simulink model "SOFC_smlkCH4"  (R2015b)
settings: Solver=ode113  SolverMode=SingleTasking  StartTime=0.0  StopTime=1000  MaxStep=1  MinStep=0.00001  RelTol=1e-3
values from neighbouring files (symbols this model uses):
  A_an = 1.05e-05    [SOFC_CH4data.m]    (also in SOFC_H2data.m)
  A_cat = 2.38e-05    [SOFC_CH4data.m]    (also in SOFC_H2data.m)
  A_cell = 180    [SOFC_begin.m]
  A_el = 0.03 / T    [SOFC_CH4data.m]    (also in SOFC_H2data.m)
  B_an = -1150    [SOFC_CH4data.m]    (also in SOFC_H2data.m)
  B_cat = 1200    [SOFC_CH4data.m]    (also in SOFC_H2data.m)
  B_el = 10300    [SOFC_CH4data.m]    (also in SOFC_H2data.m)
  c_cw = 4.18e03    (= 4180)    [SOFC_CH4data.m]    (also in SOFC_H2data.m)
  C_th = 500e03    (= 500000)    [SOFC_CH4data.m]    (also in SOFC_H2data.m)
  CV = nH2_FCin_ / n_fuel    [SOFC_CH4data.m]
  CV_H2O = nH2O_FCin_ / n_fuel    [SOFC_CH4data.m]
  E_act_an = 75e03    (= 75000)    [SOFC_CH4data.m]    (also in SOFC_H2data.m)
  E_act_cat = 96e03    (= 96000)    [SOFC_CH4data.m]    (also in SOFC_H2data.m)
  eta_ACDC = 0.90    (= 0.9)    [SOFC_CH4data.m]    (also in SOFC_H2data.m = 0.95)
  eta_comb = 0.95    [SOFC_CH4data.m]    (also in SOFC_H2data.m = 1)
  eta_hx = 0.90    (= 0.9)    [SOFC_CH4data.m]    (also in SOFC_H2data.m = 0.92)
  F = 96485    [SOFC_begin.m]
  F_airsplit = 2.0    (= 2)    [SOFC_CH4data.m]    (also in SOFC_H2data.m = 1.1)
  F_pr = 3.0711    [SOFC_CH4data.m]
  gamma_an = 5.5e4    (= 55000)    [SOFC_CH4data.m]    (also in SOFC_H2data.m)
  gamma_cat = 7.0e4    (= 70000)    [SOFC_CH4data.m]    (also in SOFC_H2data.m)
  h_airc = gamma_air * R * T / (gamma_air - 1) * ((1 / beta_c)^     ((gamma_air - 1) / gamma_air) - 1) / eta_c    [SOFC_CH4data.m]    (also in SOFC_H2data.m)
  h_airpc = (h_aircomb - h_airexh) / 1000 * M_air    [SOFC_CH4data.m]    (also in SOFC_H2data.m)
  h_airpr = (hairpr_out - hairpr_in) * M_air / eta_ph    [SOFC_CH4data.m]
  h_Arpc = (h_Arcomb - h_Arexh) / 1000 * M_Ar    [SOFC_CH4data.m]    (also in SOFC_H2data.m)
  h_CH4c = gamma_CH4 * R * T / (gamma_CH4 - 1) * ((1 / beta_c)^     ((gamma_CH4 - 1) / gamma_CH4) - 1) / eta_c    [SOFC_CH4data.m]
  h_CH4ref = -206000    [SOFC_CH4data.m]
  h_CO2pc = (h_CO2comb - h_CO2exh) / 1000 * M_CO2    [SOFC_CH4data.m]    (also in SOFC_H2data.m)
  h_cond = 500    [SOFC_CH4data.m]    (also in SOFC_H2data.m)
  h_conv = 0.1    [SOFC_CH4data.m]    (also in SOFC_H2data.m)
  h_COpc = C_COcomb * (Tcomb - Texh) * M_CO    (= 23740.08)    [SOFC_CH4data.m]
  h_fpr = (hfpr_out - hfpr_in) / eta_ph    [SOFC_CH4data.m]
  h_H2Opc = C_H2Ocomb * (Tcomb - Texh) / 1000 * M_H2O    [SOFC_CH4data.m]    (also in SOFC_H2data.m)
  h_H2Opcvap = WaterEnthalpyVaporization (pcomb/101325, Texh)    [SOFC_CH4data.m]    (also in SOFC_H2data.m)
  h_H2Opr = ((hH2Opr_out - hH2Opr_in) * M_H2O + h_H2Oprv) / eta_ph    [SOFC_CH4data.m]
  h_H2pc = C_H2comb * (Tcomb - Texh) / 1000 * M_H2    [SOFC_CH4data.m]    (also in SOFC_H2data.m)
  h_N2pc = (h_N2comb - h_N2exh) / 1000 * M_N2    [SOFC_CH4data.m]    (also in SOFC_H2data.m)
  h_O2pc = (h_O2comb - h_O2exh) / 1000 * M_O2    [SOFC_CH4data.m]    (also in SOFC_H2data.m)
  i_max = 0.88    [SOFC_CH4data.m]    (also in SOFC_H2data.m)
  K_H2 = 8.34e-01    (= 0.834)    [SOFC_CH4data.m]    (also in SOFC_H2data.m)
  K_H2O = 2.81e-01    (= 0.281)    [SOFC_CH4data.m]    (also in SOFC_H2data.m)
  K_O2 = 2.52e-00    (= 2.52)    [SOFC_CH4data.m]    (also in SOFC_H2data.m)
  K_r = N_cell / (4 * F)    [SOFC_CH4data.m]    (also in SOFC_H2data.m)
  lambda = 9.15    [SOFC_begin.m]
  m_cw = 0.25000    (= 0.25)    [SOFC_CH4data.m]    (also in SOFC_H2data.m)
  N_cell = 38    [SOFC_begin.m]
  p_atm = 1.01325e05    (= 101325)    [SOFC_begin.m]
  P_gamma = 190.0    (= 190)    [SOFC_CH4data.m]    (also in SOFC_H2data.m = 100)
  p_H20 = pp_fin(6) / 101325    [SOFC_CH4data.m]    (also in SOFC_H2data.m = y_H2in * p_an / 101325)
  p_H2O0 = pp_fin(7) / 101325    [SOFC_CH4data.m]    (also in SOFC_H2data.m = y_H2Oin * p_an / 101325)
  p_O20 = pp_ain(5) / 101325    [SOFC_CH4data.m]    (also in SOFC_H2data.m = x_O2in * p_cat / 101325)
  Q_COref = n_COref * h_COref    [SOFC_CH4data.m]
  Q_gamma = 0.0    (= 0)    [SOFC_CH4data.m]    (also in SOFC_H2data.m = 30)
  R = P_SOFC ./ (P_SOFC ./ etae_aux .* etat)    [SOFC_begin.m]
  R_th = 0.0817    [SOFC_CH4data.m]    (also in SOFC_H2data.m)
  SC = 2.16    [SOFC_CH4data.m]
  T = 750 + 273.15    (= 1023.15)    [SOFC_begin.m]
  T0 = T_a    [SOFC_CH4data.m]    (also in SOFC_H2data.m)
  T_a = 25    [SOFC_begin.m]
  t_an = 0.0545    [SOFC_CH4data.m]    (also in SOFC_H2data.m)
  t_cat = 0.004    [SOFC_CH4data.m]    (also in SOFC_H2data.m)
  T_cwin = 20 + 0    (= 20)    [SOFC_CH4data.m]    (also in SOFC_H2data.m)
  T_des = T - 273.15    [SOFC_CH4data.m]    (also in SOFC_H2data.m)
  t_el = 0.0005    [SOFC_CH4data.m]    (also in SOFC_H2data.m)
  tau1_ref = 2    [SOFC_CH4data.m]
  tau2_ref = 2    [SOFC_CH4data.m]
  tau_H2 = 26.1    [SOFC_CH4data.m]    (also in SOFC_H2data.m)
  tau_H2O = 78.30    (= 78.3)    [SOFC_CH4data.m]    (also in SOFC_H2data.m)
  tau_hx = 15.0    (= 15)    [SOFC_CH4data.m]    (also in SOFC_H2data.m)
  tau_O2 = 2.91    [SOFC_CH4data.m]    (also in SOFC_H2data.m)
  tau_ph = 5.00    (= 5)    [SOFC_CH4data.m]    (also in SOFC_H2data.m)
  tau_th = C_th * R_th    (= 40850)    [SOFC_CH4data.m]    (also in SOFC_H2data.m)
  theta = 0.910    (= 0.91)    [SOFC_CH4data.m]    (also in SOFC_H2data.m)
  U = polyval(polU, n_CH4in(1))    [SOFC_CH4data.m]    (also in SOFC_H2data.m = polyval(polU, n_H2in(1)))
  V_tn = 1.48    [SOFC_CH4data.m]    (also in SOFC_H2data.m)
  x_Ar = 0.0092    [SOFC_begin.m]
  x_CO2 = 0.0004    [SOFC_begin.m]
  x_H2O = 0.0103    [SOFC_begin.m]
  x_H2Ovap = WaterSaturationPressure (Texh) / (pcomb/101325)    [SOFC_CH4data.m]    (also in SOFC_H2data.m)
  x_N2 = 0.7728    [SOFC_begin.m]
  x_O2 = 0.2073    [SOFC_begin.m]
  xi1 = n_fuel * yy_in(1)    [SOFC_CH4data.m]    (also in SOFC_cellstack.m = n_a * yy(1))
  xi2 = n_fuel * (yy_in(1) + yy_in(2)) * 0.92    [SOFC_CH4data.m]    (also in SOFC_cellstack.m = xi)
  xi3 = U * n_fuel * (4 * yy_in(1) + yy_in(2) + yy_in(6))    [SOFC_CH4data.m]    (also in SOFC_cellstack.m = U * n_a * (4 * yy(1) + yy(2) + yy(6)))
  xi4 = nn_fout(6) * eta_comb    [SOFC_CH4data.m]    (also in SOFC_H2data.m = n_H2out * eta_comb)
  xi5 = nn_fout(2) * eta_comb    [SOFC_CH4data.m]
  y_CH4 = 0.2832    [SOFC_begin.m]
  y_CO = 0.0207    [SOFC_begin.m]
  y_CO2 = 0    [SOFC_begin.m]
  y_H2 = 0.0482    [SOFC_begin.m]
  y_H2O = 0.6348    [SOFC_begin.m]
  y_N2 = 0.0131    [SOFC_begin.m]
undefined symbols (not defined in the file or in its folder): magnitude
settings Model: Creator=gapaolo  LastModifiedBy=gapaolo
settings DataIOCC: SaveFormat=Array
settings OptimizationCC: BlockReduction=off  BooleanDataType=off
settings DebuggingCC: AlgebraicLoopMsg=none  SaveWithParameterizedLinksMsg=none  UnderspecifiedInitializationDetection=Classic  MergeDetectMultiDrivingBlocksExec=none  SignalResolutionControl=TryResolveAllWithWarning
settings HardwareCC: ProdBitPerPointer=32  ProdLargestAtomicFloat=None  ProdIntDivRoundTo=Undefined  ProdEndianess=Unspecified  ProdWordSize=32  ProdHWDeviceType=32-bit Generic  TargetUnknown=on
settings GRTTargetCC: GeneratePreprocessorConditionals=Disable all
settings ConfigComp: CovModelRefEnable=Off  CovSFcnEnable=off

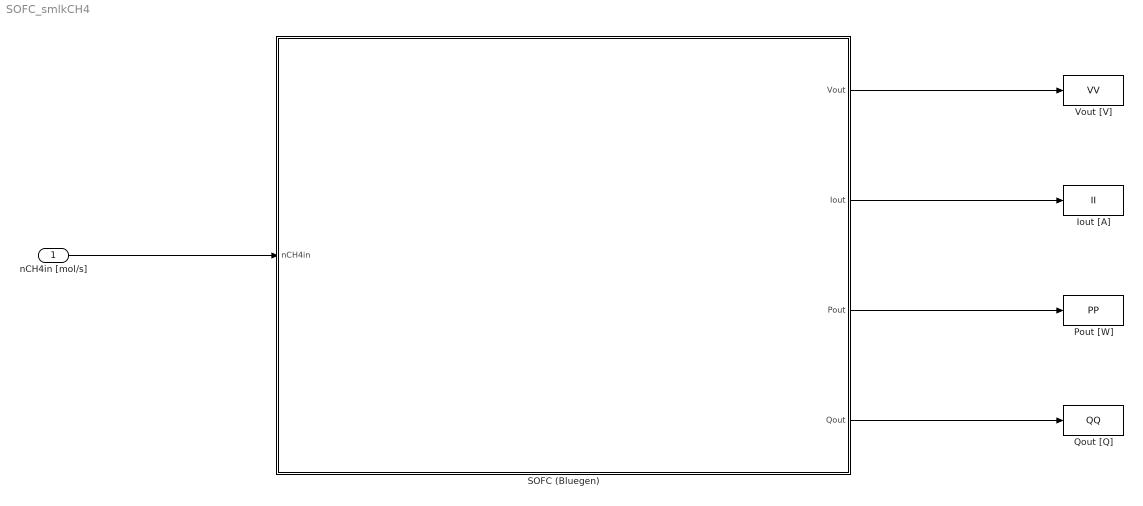
== system SOFC_smlkCH4 ==
  nCH4in [mol/s] : Inport
  Iout [A] : ToWorkspace  VariableName=II  SaveFormat=Timeseries  SampleTime=-1
  Pout [W] : ToWorkspace  VariableName=PP  SaveFormat=Timeseries  SampleTime=-1
  Qout [Q] : ToWorkspace  VariableName=QQ  SaveFormat=Timeseries  SampleTime=-1
  SOFC (Bluegen) : Subsystem
  Vout [V] : ToWorkspace  VariableName=VV  SaveFormat=Timeseries  SampleTime=-1
  wires:
  nCH4in [mol/s]/1 -> SOFC (Bluegen)/1(nCH4in)
  SOFC (Bluegen)/1(Vout) -> Vout [V]/1
  SOFC (Bluegen)/2(Iout) -> Iout [A]/1
  SOFC (Bluegen)/3(Pout) -> Pout [W]/1
  SOFC (Bluegen)/4(Qout) -> Qout [Q]/1

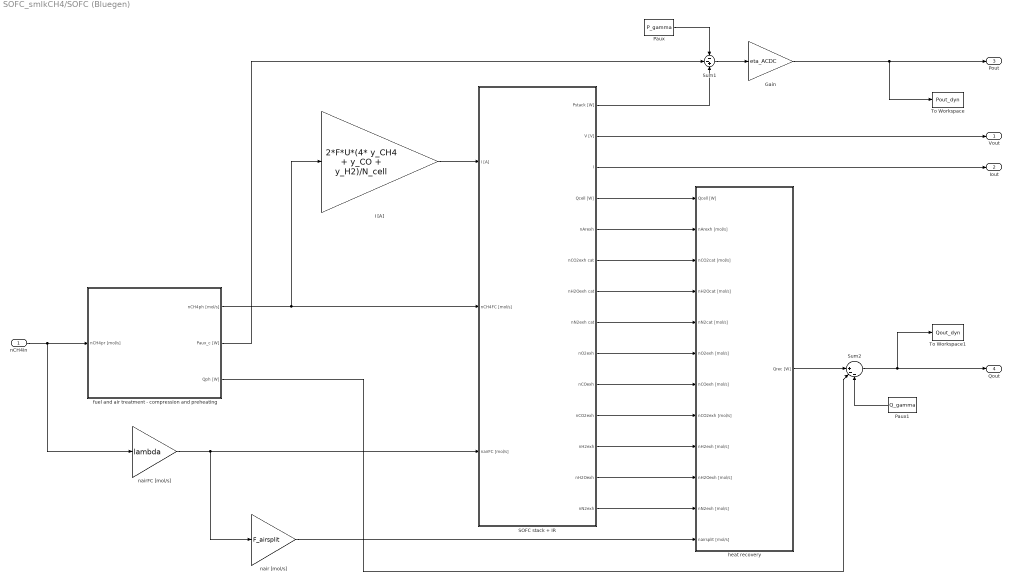
== system SOFC_smlkCH4/SOFC (Bluegen) ==
  nCH4in : Inport
  Gain : Gain  Gain=eta_ACDC
  I [A] : Gain  Gain=2*F*U*(4* y_CH4 + y_CO + y_H2)/N_cell
  Paux : Constant  Value=P_gamma
  Paux1 : Constant  Value=Q_gamma
  SOFC stack + IR : Subsystem
  Sum1 : Sum  Inputs=--+
  Sum2 : Sum  Inputs=||+--
  To Workspace : ToWorkspace  VariableName=Pout_dyn  SaveFormat=Timeseries  SampleTime=-1
  To Workspace1 : ToWorkspace  VariableName=Qout_dyn  SaveFormat=Timeseries  SampleTime=-1
  fuel and air treatment - compression and preheating : Subsystem
  heat recovery : Subsystem
  nair [mol/s] : Gain  Gain=F_airsplit
  nairFC [mol/s] : Gain  Gain=lambda
  Vout : Outport
  Iout : Outport  Port=2
  Pout : Outport  Port=3
  Qout : Outport  Port=4
  wires:
  nCH4in/1 -> fuel and air treatment - compression and preheating/1(nCH4pr [mol/s]), nairFC [mol/s]/1
  fuel and air treatment - compression and preheating/1(nCH4ph [mol/s]) -> I [A]/1, SOFC stack + IR/2(nCH4FC [mol/s])
  I [A]/1 -> SOFC stack + IR/1(I [A])
  nairFC [mol/s]/1 -> nair [mol/s]/1, SOFC stack + IR/3(nairFC [mol/s])
  SOFC stack + IR/4(Qcell [W]) -> heat recovery/1(Qcell [W])
  SOFC stack + IR/5(nArexh) -> heat recovery/2(nArexh [mol/s])
  SOFC stack + IR/6(nCO2exh cat) -> heat recovery/3(nCO2cat [mol/s])
  SOFC stack + IR/7(nH2Oexh cat) -> heat recovery/4(nH2Ocat [mol/s])
  SOFC stack + IR/8(nN2exh cat) -> heat recovery/5(nN2cat [mol/s])
  SOFC stack + IR/9(nO2exh) -> heat recovery/6(nO2exh [mol/s])
  SOFC stack + IR/11(nCO2exh) -> heat recovery/8(nCO2exh [mol/s])
  SOFC stack + IR/12(nH2exh) -> heat recovery/9(nH2exh [mol/s])
  SOFC stack + IR/13(nH2Oexh) -> heat recovery/10(nH2Oexh [mol/s])
  nair [mol/s]/1 -> heat recovery/12(nairsplit [mol/s])
  SOFC stack + IR/10(nCOexh) -> heat recovery/7(nCOexh [mol/s])
  SOFC stack + IR/14(nN2exh) -> heat recovery/11(nN2exh [mol/s])
  SOFC stack + IR/2(V [V]) -> Vout/1
  SOFC stack + IR/3("I ") -> Iout/1
  Sum1/1 -> Gain/1
  SOFC stack + IR/1(Pstack [W]) -> Sum1/3
  fuel and air treatment - compression and preheating/2(Paux_c [W]) -> Sum1/2
  Paux/1 -> Sum1/1
  heat recovery/1(Qrec [W]) -> Sum2/1
  Sum2/1 -> Qout/1, To Workspace1/1
  Gain/1 -> To Workspace/1, Pout/1
  fuel and air treatment - compression and preheating/3(Qph [W]) -> Sum2/2
  Paux1/1 -> Sum2/3

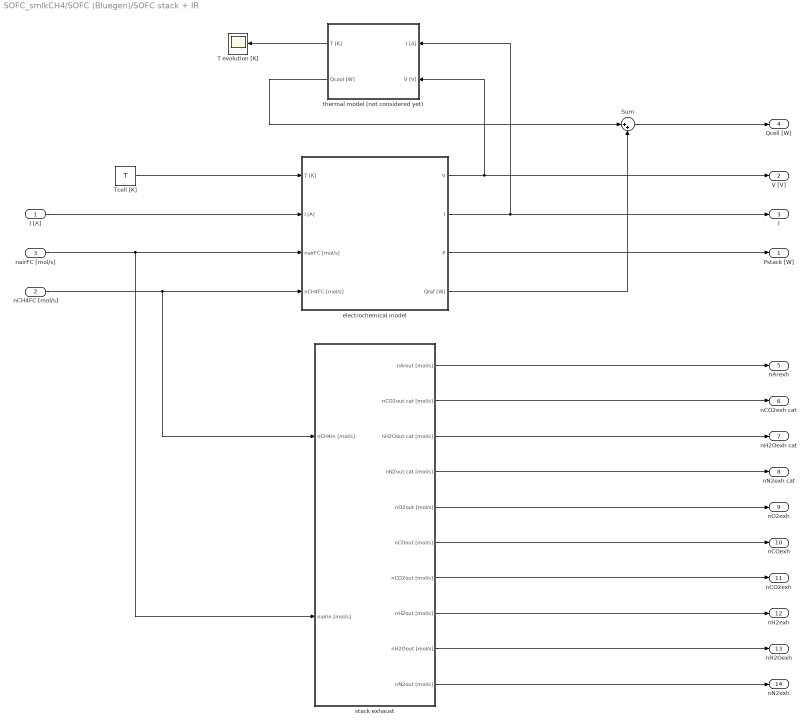
== system SOFC_smlkCH4/SOFC (Bluegen)/SOFC stack + IR ==
  I [A] : Inport
  nCH4FC [mol/s] : Inport  Port=2
  nairFC [mol/s] : Inport  Port=3
  Sum : Sum  Inputs=|++
  T evolution [K] : Scope
  Tcell [K] : Constant  Value=T
  electrochemical model : Subsystem
  stack exhaust : Subsystem
  thermal model (not considered yet) : Subsystem
  Pstack [W] : Outport
  V [V] : Outport  Port=2
  "I " : Outport  Port=3
  Qcell [W] : Outport  Port=4
  nArexh : Outport  Port=5
  nCO2exh cat : Outport  Port=6
  nH2Oexh cat : Outport  Port=7
  nN2exh cat : Outport  Port=8
  nO2exh : Outport  Port=9
  nCOexh : Outport  Port=10
  nCO2exh : Outport  Port=11
  nH2exh : Outport  Port=12
  nH2Oexh : Outport  Port=13
  nN2exh : Outport  Port=14
  wires:
  I [A]/1 -> electrochemical model/2(I [A])
  nairFC [mol/s]/1 -> stack exhaust/2(nairin [mol/s]), electrochemical model/3(nairFC [mol/s])
  nCH4FC [mol/s]/1 -> stack exhaust/1(nCH4in [mol/s]), electrochemical model/4(nCH4FC [mol/s])
  electrochemical model/1(V) -> thermal model (not considered yet)/2(V [V]), V [V]/1
  electrochemical model/2(I) -> "I "/1, thermal model (not considered yet)/1(I [A])
  thermal model (not considered yet)/1(T [K]) -> T evolution [K]/1
  thermal model (not considered yet)/2(Qcool [W]) -> Sum/1
  electrochemical model/3(P) -> Pstack [W]/1
  Tcell [K]/1 -> electrochemical model/1(T [K])
  electrochemical model/4(Qref [W]) -> Sum/2
  Sum/1 -> Qcell [W]/1
  stack exhaust/10(nN2out [mol/s]) -> nN2exh/1
  stack exhaust/9(nH2Oout [mol/s]) -> nH2Oexh/1
  stack exhaust/8(nH2out [mol/s]) -> nH2exh/1
  stack exhaust/7(nCO2out [mol/s]) -> nCO2exh/1
  stack exhaust/6(nCOout [mol/s]) -> nCOexh/1
  stack exhaust/5(nO2out [mol/s]) -> nO2exh/1
  stack exhaust/4(nN2out cat [mol/s]) -> nN2exh cat/1
  stack exhaust/3(nH2Oout cat [mol/s]) -> nH2Oexh cat/1
  stack exhaust/2(nCO2out cat [mol/s]) -> nCO2exh cat/1
  stack exhaust/1(nArout [mol/s]) -> nArexh/1

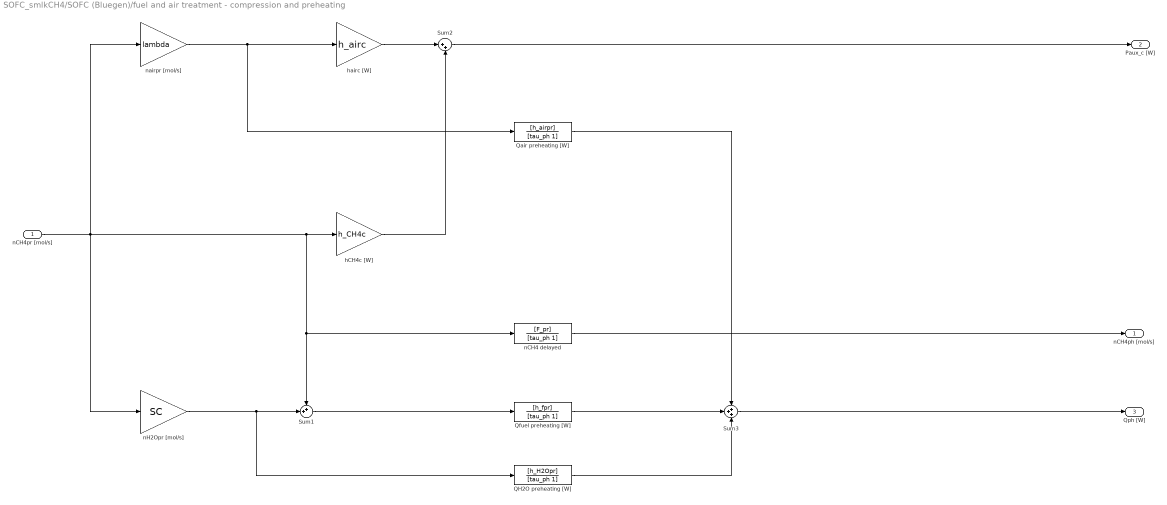
== system SOFC_smlkCH4/SOFC (Bluegen)/fuel and air treatment - compression and preheating ==
  nCH4pr [mol/s] : Inport
  QH2O preheating [W] : TransferFcn  Numerator=[h_H2Opr]  Denominator=[tau_ph 1]
  Qair preheating [W] : TransferFcn  Numerator=[h_airpr]  Denominator=[tau_ph 1]
  Qfuel preheating [W] : TransferFcn  Numerator=[h_fpr]  Denominator=[tau_ph 1]
  Sum1 : Sum  Inputs=++|
  Sum2 : Sum  Inputs=|++
  Sum3 : Sum  Inputs=+++
  hCH4c [W] : Gain  Gain=h_CH4c
  hairc [W] : Gain  Gain=h_airc
  nCH4 delayed : TransferFcn  Numerator=[F_pr]  Denominator=[tau_ph 1]
  nH2Opr [mol/s] : Gain  Gain=SC
  nairpr [mol/s] : Gain  Gain=lambda
  nCH4ph [mol/s] : Outport
  Paux_c [W] : Outport  Port=2
  Qph [W] : Outport  Port=3
  wires:
  nCH4pr [mol/s]/1 -> hCH4c [W]/1, nCH4 delayed/1, Sum1/1, nairpr [mol/s]/1, nH2Opr [mol/s]/1
  nH2Opr [mol/s]/1 -> QH2O preheating [W]/1, Sum1/2
  nairpr [mol/s]/1 -> Qair preheating [W]/1, hairc [W]/1
  hairc [W]/1 -> Sum2/1
  hCH4c [W]/1 -> Sum2/2
  Sum2/1 -> Paux_c [W]/1
  Sum1/1 -> Qfuel preheating [W]/1
  Qfuel preheating [W]/1 -> Sum3/2
  QH2O preheating [W]/1 -> Sum3/3
  Sum3/1 -> Qph [W]/1
  nCH4 delayed/1 -> nCH4ph [mol/s]/1
  Qair preheating [W]/1 -> Sum3/1

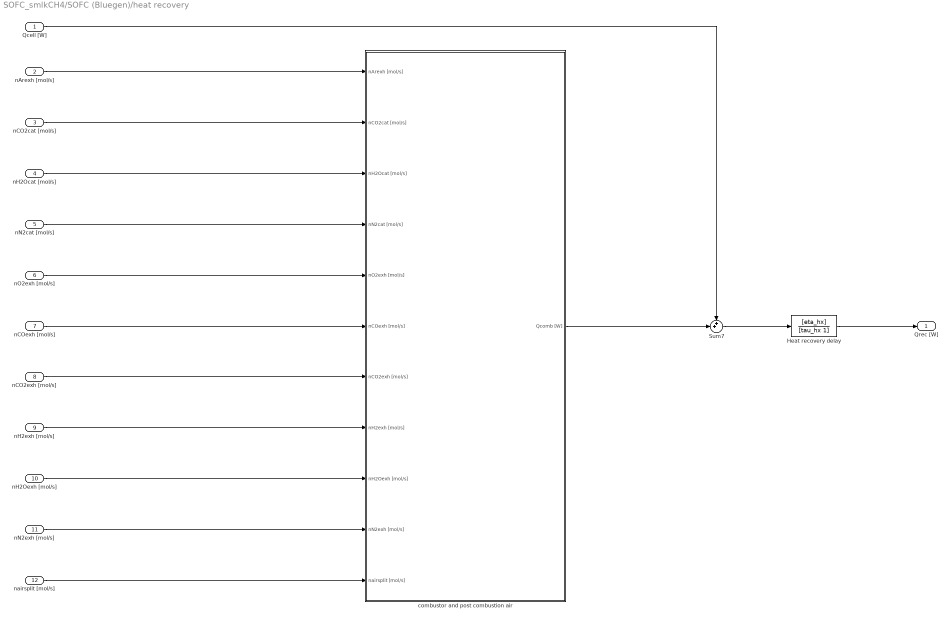
== system SOFC_smlkCH4/SOFC (Bluegen)/heat recovery ==
  Qcell [W] : Inport
  nArexh [mol/s] : Inport  Port=2
  nCO2cat [mol/s] : Inport  Port=3
  nH2Ocat [mol/s] : Inport  Port=4
  nN2cat [mol/s] : Inport  Port=5
  nO2exh [mol/s] : Inport  Port=6
  nCOexh [mol/s] : Inport  Port=7
  nCO2exh [mol/s] : Inport  Port=8
  nH2exh [mol/s] : Inport  Port=9
  nH2Oexh [mol/s] : Inport  Port=10
  nN2exh [mol/s] : Inport  Port=11
  nairsplit [mol/s] : Inport  Port=12
  Heat recovery delay : TransferFcn  Numerator=[eta_hx]  Denominator=[tau_hx 1]
  Sum7 : Sum  Inputs=++|
  combustor and post combustion air : Subsystem
  Qrec [W] : Outport
  wires:
  Heat recovery delay/1 -> Qrec [W]/1
  nArexh [mol/s]/1 -> combustor and post combustion air/1(nArexh [mol/s])
  nCO2cat [mol/s]/1 -> combustor and post combustion air/2(nCO2cat [mol/s])
  nH2Ocat [mol/s]/1 -> combustor and post combustion air/3(nH2Ocat [mol/s])
  nN2cat [mol/s]/1 -> combustor and post combustion air/4(nN2cat [mol/s])
  nO2exh [mol/s]/1 -> combustor and post combustion air/5(nO2exh [mol/s])
  nCOexh [mol/s]/1 -> combustor and post combustion air/6(nCOexh [mol/s])
  nCO2exh [mol/s]/1 -> combustor and post combustion air/7(nCO2exh [mol/s])
  nH2exh [mol/s]/1 -> combustor and post combustion air/8(nH2exh [mol/s])
  nH2Oexh [mol/s]/1 -> combustor and post combustion air/9(nH2Oexh [mol/s])
  nN2exh [mol/s]/1 -> combustor and post combustion air/10(nN2exh [mol/s])
  nairsplit [mol/s]/1 -> combustor and post combustion air/11(nairsplit [mol/s])
  combustor and post combustion air/1(Qcomb [W]) -> Sum7/2
  Sum7/1 -> Heat recovery delay/1
  Qcell [W]/1 -> Sum7/1

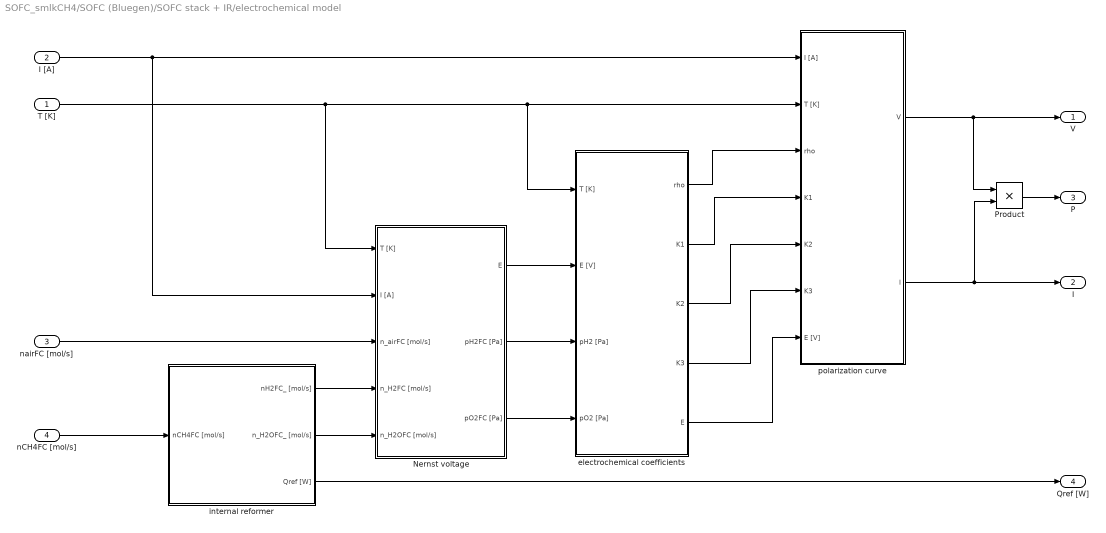
== system SOFC_smlkCH4/SOFC (Bluegen)/SOFC stack + IR/electrochemical model ==
  T [K] : Inport
  I [A] : Inport  Port=2
  nairFC [mol/s] : Inport  Port=3
  nCH4FC [mol/s] : Inport  Port=4
  Nernst voltage : Subsystem
  Product : Product
  electrochemical coefficients : Subsystem
  internal reformer : Subsystem
  polarization curve : Subsystem
  V : Outport
  I : Outport  Port=2
  P : Outport  Port=3
  Qref [W] : Outport  Port=4
  wires:
  internal reformer/1(nH2FC_ [mol/s]) -> Nernst voltage/4(n_H2FC [mol/s])
  nairFC [mol/s]/1 -> Nernst voltage/3(n_airFC [mol/s])
  T [K]/1 -> Nernst voltage/1(T [K]), polarization curve/2(T [K]), electrochemical coefficients/1(T [K])
  internal reformer/2(n_H2OFC_ [mol/s]) -> Nernst voltage/5(n_H2OFC [mol/s])
  nCH4FC [mol/s]/1 -> internal reformer/1(nCH4FC [mol/s])
  I [A]/1 -> Nernst voltage/2(I [A]), polarization curve/1("I [A] ")
  Nernst voltage/2(pH2FC [Pa]) -> electrochemical coefficients/3("pH2 [Pa] ")
  Nernst voltage/3(pO2FC [Pa]) -> electrochemical coefficients/4(pO2 [Pa])
  Nernst voltage/1(E) -> electrochemical coefficients/2(E [V])
  electrochemical coefficients/1(rho) -> polarization curve/3(rho)
  electrochemical coefficients/2(K1) -> polarization curve/4(K1)
  electrochemical coefficients/3(K2) -> polarization curve/5(K2)
  electrochemical coefficients/4(K3) -> polarization curve/6(K3)
  electrochemical coefficients/5(E) -> polarization curve/7(E [V])
  polarization curve/2(I) -> Product/2, I/1
  polarization curve/1(V) -> Product/1, V/1
  Product/1 -> P/1
  internal reformer/3(Qref [W]) -> Qref [W]/1

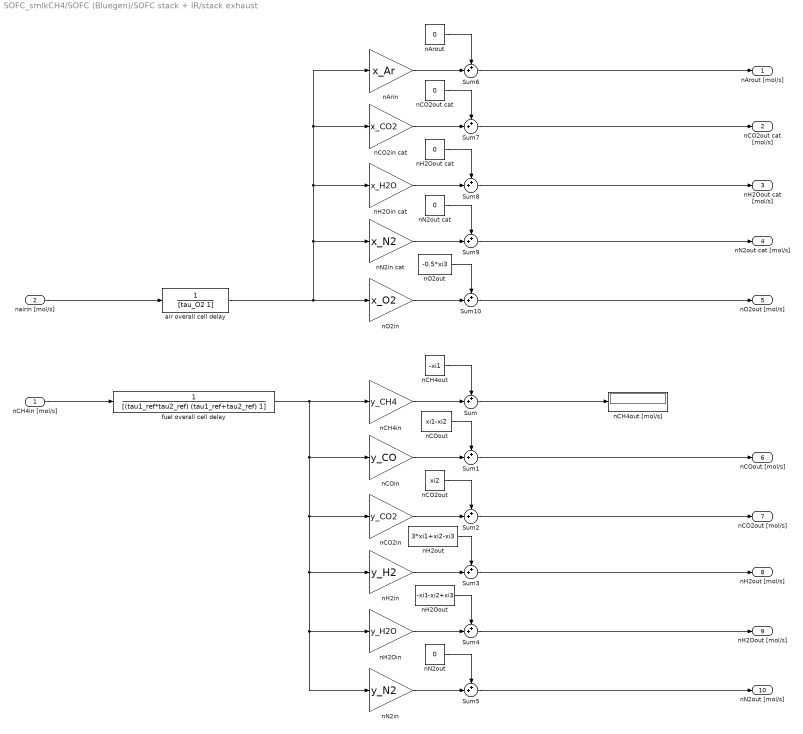
== system SOFC_smlkCH4/SOFC (Bluegen)/SOFC stack + IR/stack exhaust ==
  nCH4in [mol/s] : Inport
  nairin [mol/s] : Inport  Port=2
  Sum{,1..10} (11 alike) : Sum  Inputs=++|
  air overall cell delay : TransferFcn  Denominator=[tau_O2 1]  ContinuousStateAttributes='p_O2'
  fuel overall cell delay : TransferFcn  Denominator=[(tau1_ref*tau2_ref) (tau1_ref+tau2_ref) 1]  ContinuousStateAttributes='q_H2'
  nArin : Gain  Gain=x_Ar
  nArout : Constant  Value=0
  nCH4in : Gain  Gain=y_CH4
  nCH4out : Constant  Value=-xi1
  nCH4out [mol/s] : Display
  nCO2in : Gain  Gain=y_CO2
  nCO2in cat : Gain  Gain=x_CO2
  nCO2out : Constant  Value=xi2
  nCO2out cat : Constant  Value=0
  nCOin : Gain  Gain=y_CO
  nCOout : Constant  Value=xi1-xi2
  nH2Oin : Gain  Gain=y_H2O
  nH2Oin cat : Gain  Gain=x_H2O
  nH2Oout : Constant  Value=-xi1-xi2+xi3
  nH2Oout cat : Constant  Value=0
  nH2in : Gain  Gain=y_H2
  nH2out : Constant  Value=3*xi1+xi2-xi3
  nN2in : Gain  Gain=y_N2
  nN2in cat : Gain  Gain=x_N2
  nN2out : Constant  Value=0
  nN2out cat : Constant  Value=0
  nO2in : Gain  Gain=x_O2
  nO2out : Constant  Value=-0.5*xi3
  nArout [mol/s] : Outport
  nCO2out cat [mol/s] : Outport  Port=2
  nH2Oout cat [mol/s] : Outport  Port=3
  nN2out cat [mol/s] : Outport  Port=4
  nO2out [mol/s] : Outport  Port=5
  nCOout [mol/s] : Outport  Port=6
  nCO2out [mol/s] : Outport  Port=7
  nH2out [mol/s] : Outport  Port=8
  nH2Oout [mol/s] : Outport  Port=9
  nN2out [mol/s] : Outport  Port=10
  wires:
  nCH4in [mol/s]/1 -> fuel overall cell delay/1
  nairin [mol/s]/1 -> air overall cell delay/1
  fuel overall cell delay/1 -> nN2in/1, nH2Oin/1, nH2in/1, nCO2in/1, nCOin/1, nCH4in/1
  nCH4in/1 -> Sum/2
  nCH4out/1 -> Sum/1
  nCOin/1 -> Sum1/2
  nCOout/1 -> Sum1/1
  nCO2in/1 -> Sum2/2
  nCO2out/1 -> Sum2/1
  nH2in/1 -> Sum3/2
  nH2out/1 -> Sum3/1
  nH2Oin/1 -> Sum4/2
  nH2Oout/1 -> Sum4/1
  nN2in/1 -> Sum5/2
  nN2out/1 -> Sum5/1
  nArin/1 -> Sum6/2
  nArout/1 -> Sum6/1
  nCO2in cat/1 -> Sum7/2
  nCO2out cat/1 -> Sum7/1
  nH2Oin cat/1 -> Sum8/2
  nH2Oout cat/1 -> Sum8/1
  nN2in cat/1 -> Sum9/2
  nN2out cat/1 -> Sum9/1
  nO2in/1 -> Sum10/2
  nO2out/1 -> Sum10/1
  air overall cell delay/1 -> nH2Oin cat/1, nCO2in cat/1, nArin/1, nN2in cat/1, nO2in/1
  Sum6/1 -> nArout [mol/s]/1
  Sum7/1 -> nCO2out cat [mol/s]/1
  Sum8/1 -> nH2Oout cat [mol/s]/1
  Sum9/1 -> nN2out cat [mol/s]/1
  Sum10/1 -> nO2out [mol/s]/1
  Sum4/1 -> nH2Oout [mol/s]/1
  Sum3/1 -> nH2out [mol/s]/1
  Sum5/1 -> nN2out [mol/s]/1
  Sum2/1 -> nCO2out [mol/s]/1
  Sum1/1 -> nCOout [mol/s]/1
  Sum/1 -> nCH4out [mol/s]/1

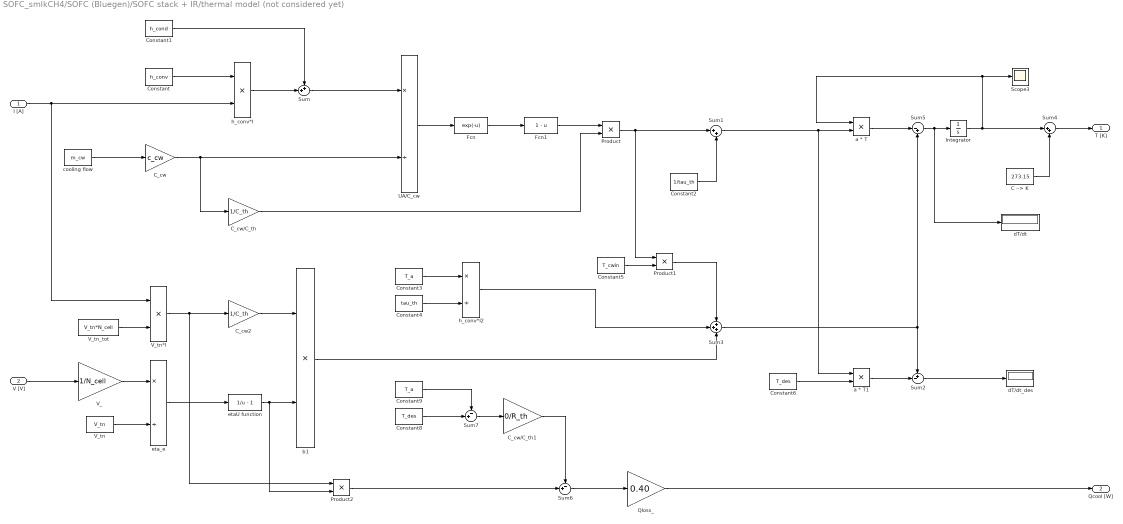
== system SOFC_smlkCH4/SOFC (Bluegen)/SOFC stack + IR/thermal model (not considered yet) ==
  I [A] : Inport
  V [V] : Inport  Port=2
  C --> K : Constant  Value=273.15
  C_cw : Gain  Gain=c_cw
  C_cw/C_th : Gain  Gain=1/C_th
  C_cw/C_th1 : Gain  Gain=0/R_th
  C_cw2 : Gain  Gain=1/C_th
  Constant : Constant  Value=h_conv
  Constant1 : Constant  Value=h_cond
  Constant2 : Constant  Value=1/tau_th
  Constant3 : Constant  Value=T_a
  Constant4 : Constant  Value=tau_th
  Constant5 : Constant  Value=T_cwin
  Constant6 : Constant  Value=T_des
  Constant8 : Constant  Value=T_des
  Constant9 : Constant  Value=T_a
  Fcn : Fcn  Expr=exp(-u)
  Fcn1 : Fcn  Expr=1 - u
  Integrator : Integrator  InitialCondition=T0  AbsoluteTolerance=1e-6
  Product : Product
  Product1 : Product
  Product2 : Product
  Qloss_ : Gain  Gain=0.40
  Scope3 : Scope
  Sum : Sum  Inputs=++|
  Sum1 : Sum  Inputs=|++
  Sum2 : Sum  Inputs=+-|
  Sum3 : Sum  Inputs=+++
  Sum4 : Sum  Inputs=|++
  Sum5 : Sum  Inputs=|-+
  Sum6 : Sum  Inputs=-+|
  Sum7 : Sum  Inputs=-+|
  UA/C_cw : Product  Inputs=*/
  V_ : Gain  Gain=1/N_cell
  V_tn : Constant  Value=V_tn
  V_tn*I : Product
  V_tn_tot : Constant  Value=V_tn*N_cell
  a * T : Product
  a * T1 : Product
  b1 : Product
  cooling flow : Constant  Value=m_cw
  dT/dt : Display
  dT/dt_des : Display
  etaU function : Fcn  Expr=1/u - 1
  eta_e : Product  Inputs=*/
  h_conv*I : Product
  h_conv*I2 : Product  Inputs=*/
  T [K] : Outport
  Qcool [W] : Outport  Port=2
  wires:
  V_tn_tot/1 -> V_tn*I/2
  eta_e/1 -> etaU function/1
  V_tn/1 -> eta_e/2
  V_/1 -> eta_e/1
  b1/1 -> Sum3/3
  h_conv*I2/1 -> Sum3/2
  Product1/1 -> Sum3/1
  Constant5/1 -> Product1/2
  Constant4/1 -> h_conv*I2/2
  Constant3/1 -> h_conv*I2/1
  C_cw2/1 -> b1/1
  V [V]/1 -> V_/1
  Constant2/1 -> Sum1/2
  Product/1 -> Sum1/1, Product1/1
  C_cw/C_th/1 -> Product/2
  Fcn1/1 -> Product/1
  C_cw/1 -> C_cw/C_th/1, UA/C_cw/2
  Fcn/1 -> Fcn1/1
  UA/C_cw/1 -> Fcn/1
  cooling flow/1 -> C_cw/1
  Sum/1 -> UA/C_cw/1
  Constant1/1 -> Sum/1
  h_conv*I/1 -> Sum/2
  Constant/1 -> h_conv*I/1
  I [A]/1 -> h_conv*I/2, V_tn*I/1
  Integrator/1 -> Sum4/1, a * T/1, Scope3/1
  a * T/1 -> Sum5/1
  Sum3/1 -> Sum5/2, Sum2/1
  Sum1/1 -> a * T1/1, a * T/2
  Constant6/1 -> a * T1/2
  a * T1/1 -> Sum2/2
  Sum2/1 -> dT/dt_des/1
  C --> K/1 -> Sum4/2
  Sum4/1 -> T [K]/1
  Product2/1 -> Sum6/2
  Constant8/1 -> Sum7/2
  Constant9/1 -> Sum7/1
  Sum7/1 -> C_cw/C_th1/1
  C_cw/C_th1/1 -> Sum6/1
  V_tn*I/1 -> Product2/1, C_cw2/1
  etaU function/1 -> Product2/2, b1/2
  Sum5/1 -> dT/dt/1, Integrator/1
  Sum6/1 -> Qloss_/1
  Qloss_/1 -> Qcool [W]/1

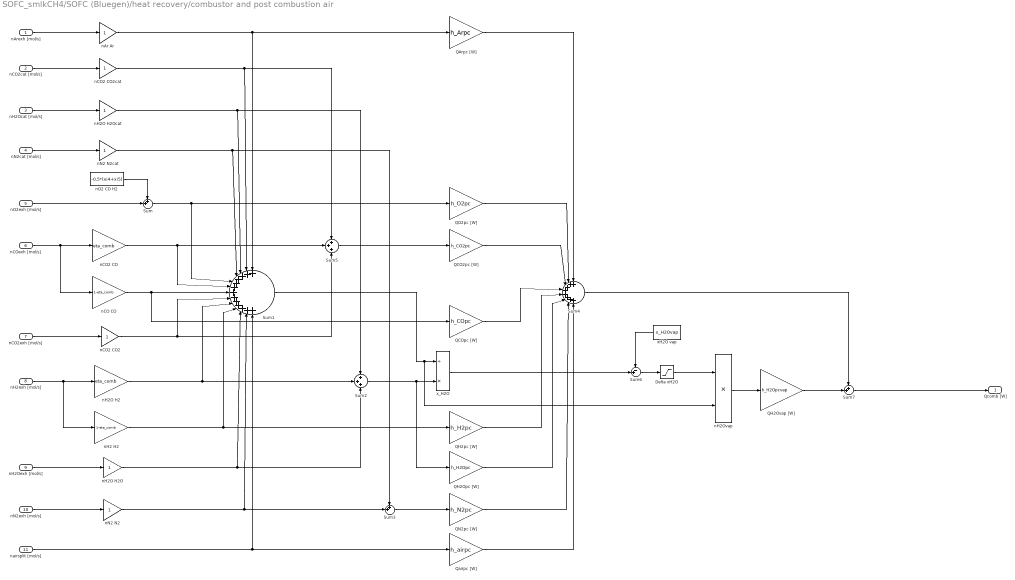
== system SOFC_smlkCH4/SOFC (Bluegen)/heat recovery/combustor and post combustion air ==
  nArexh [mol/s] : Inport
  nCO2cat [mol/s] : Inport  Port=2
  nH2Ocat [mol/s] : Inport  Port=3
  nN2cat [mol/s] : Inport  Port=4
  nO2exh [mol/s] : Inport  Port=5
  nCOexh [mol/s] : Inport  Port=6
  nCO2exh [mol/s] : Inport  Port=7
  nH2exh [mol/s] : Inport  Port=8
  nH2Oexh [mol/s] : Inport  Port=9
  nN2exh [mol/s] : Inport  Port=10
  nairsplit [mol/s] : Inport  Port=11
  Delta xH2O : Saturate  UpperLimit=1  LowerLimit=0
  QArpc [W] : Gain  Gain=h_Arpc
  QCO2pc [W] : Gain  Gain=h_CO2pc
  QCOpc [W] : Gain  Gain=h_COpc
  QH2Opc [W] : Gain  Gain=h_H2Opc
  QH2Ovap [W] : Gain  Gain=h_H2Opcvap
  QH2pc [W] : Gain  Gain=h_H2pc
  QN2pc [W] : Gain  Gain=h_N2pc
  QO2pc [W] : Gain  Gain=h_O2pc
  Qairpc [W] : Gain  Gain=h_airpc
  Sum : Sum  Inputs=++|
  Sum1 : Sum  Inputs=+++++++++++++
  Sum2 : Sum  Inputs=+++
  Sum3 : Sum  Inputs=++|
  Sum4 : Sum  Inputs=++++++++
  Sum5 : Sum  Inputs=+++
  Sum6 : Sum  Inputs=-+|
  Sum7 : Sum  Inputs=++|
  nAr Ar : Gain
  nCO CO : Gain  Gain=1-eta_comb
  nCO2 CO : Gain  Gain=eta_comb
  nCO2 CO2 : Gain
  nCO2 CO2cat : Gain
  nH2 H2 : Gain  Gain=1-eta_comb
  nH2O H2 : Gain  Gain=eta_comb
  nH2O H2O : Gain
  nH2O H2Ocat : Gain
  nH2Ovap : Product  Inputs=**
  nN2 N2 : Gain
  nN2 N2cat : Gain
  nO2 CO H2 : Constant  Value=-0.5*(xi4+xi5)
  xH2O vap : Constant  Value=x_H2Ovap
  x_H2O : Product  Inputs=/*
  Qcomb [W] : Outport
  wires:
  Delta xH2O/1 -> nH2Ovap/1
  QCO2pc [W]/1 -> Sum4/3
  QO2pc [W]/1 -> Sum4/2
  x_H2O/1 -> Sum6/2
  Sum5/1 -> QCO2pc [W]/1
  Sum3/1 -> QN2pc [W]/1
  QH2Opc [W]/1 -> Sum4/6
  QArpc [W]/1 -> Sum4/1
  Qairpc [W]/1 -> Sum4/8
  QN2pc [W]/1 -> Sum4/7
  nH2Ovap/1 -> QH2Ovap [W]/1
  Sum6/1 -> Delta xH2O/1
  Sum1/1 -> nH2Ovap/2, x_H2O/1
  QH2pc [W]/1 -> Sum4/5
  QCOpc [W]/1 -> Sum4/4
  xH2O vap/1 -> Sum6/1
  QH2Ovap [W]/1 -> Sum7/2
  Sum7/1 -> Qcomb [W]/1
  nArexh [mol/s]/1 -> nAr Ar/1
  nCO2cat [mol/s]/1 -> nCO2 CO2cat/1
  nH2Ocat [mol/s]/1 -> nH2O H2Ocat/1
  nN2cat [mol/s]/1 -> nN2 N2cat/1
  nO2exh [mol/s]/1 -> Sum/2
  nO2 CO H2/1 -> Sum/1
  nCOexh [mol/s]/1 -> nCO CO/1, nCO2 CO/1
  nCO2exh [mol/s]/1 -> nCO2 CO2/1
  nH2exh [mol/s]/1 -> nH2 H2/1, nH2O H2/1
  nH2Oexh [mol/s]/1 -> nH2O H2O/1
  nN2exh [mol/s]/1 -> nN2 N2/1
  nCO2 CO2/1 -> Sum1/8, Sum5/3
  nCO CO/1 -> QCOpc [W]/1, Sum1/7
  nairsplit [mol/s]/1 -> Sum1/13, Qairpc [W]/1
  nN2 N2/1 -> Sum1/12, Sum3/2
  nH2O H2O/1 -> Sum2/3, Sum1/11
  nH2 H2/1 -> Sum1/10, QH2pc [W]/1
  nH2O H2/1 -> Sum1/9, Sum2/2
  nCO2 CO/1 -> Sum5/2, Sum1/6
  Sum/1 -> Sum1/5, QO2pc [W]/1
  nN2 N2cat/1 -> Sum3/1, Sum1/4
  nCO2 CO2cat/1 -> Sum5/1, Sum1/2
  nAr Ar/1 -> QArpc [W]/1, Sum1/1
  nH2O H2Ocat/1 -> Sum2/1, Sum1/3
  Sum2/1 -> QH2Opc [W]/1, x_H2O/2
  Sum4/1 -> Sum7/1

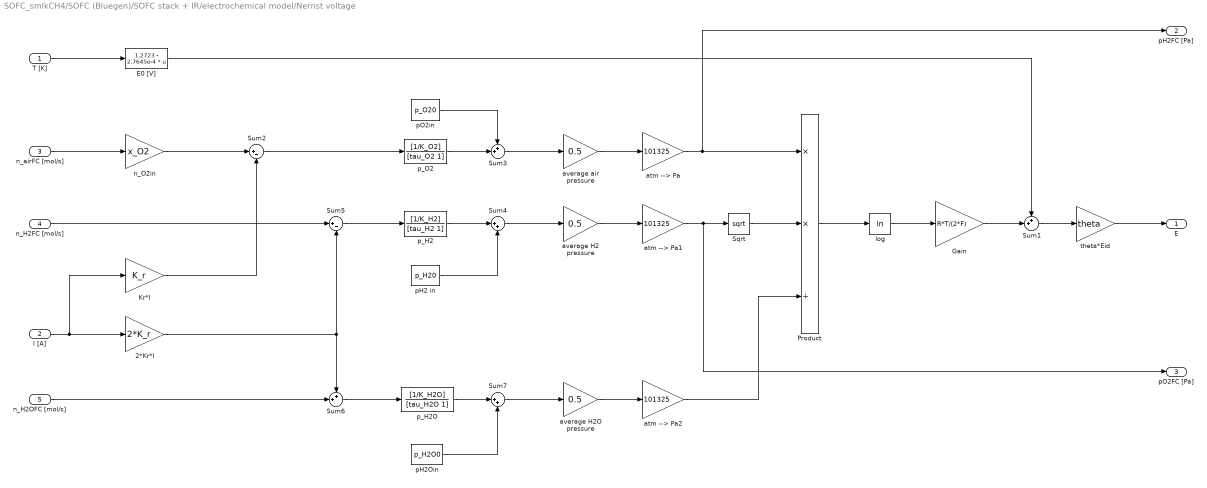
== system SOFC_smlkCH4/SOFC (Bluegen)/SOFC stack + IR/electrochemical model/Nernst voltage ==
  T [K] : Inport
  I [A] : Inport  Port=2
  n_airFC [mol/s] : Inport  Port=3
  n_H2FC [mol/s] : Inport  Port=4
  n_H2OFC [mol/s] : Inport  Port=5
  2*Kr*I : Gain  Gain=2*K_r
  E0 [V] : Fcn  Expr=1.2723 - 2.7645e-4 * u
  Gain : Gain  Gain=R*T/(2*F)
  Kr*I : Gain  Gain=K_r
  Product : Product  Inputs=**/
  Sqrt : Sqrt  SaturateOnIntegerOverflow=on
  Sum1 : Sum  Inputs=++|
  Sum2 : Sum  Inputs=|+-
  Sum3 : Sum  Inputs=++|
  Sum4 : Sum  Inputs=|++
  Sum5 : Sum  Inputs=|+-
  Sum6 : Sum  Inputs=++|
  Sum7 : Sum  Inputs=|++
  atm --> Pa : Gain  Gain=101325
  atm --> Pa1 : Gain  Gain=101325
  atm --> Pa2 : Gain  Gain=101325
  average H2 pressure : Gain  Gain=0.5
  average H2O pressure : Gain  Gain=0.5
  average air pressure : Gain  Gain=0.5
  log : Math  Operator=log  SaturateOnIntegerOverflow=on
  n_O2in : Gain  Gain=x_O2
  pH2 in : Constant  Value=p_H20
  pH2Oin : Constant  Value=p_H2O0
  pO2in : Constant  Value=p_O20
  p_H2 : TransferFcn  Numerator=[1/K_H2]  Denominator=[tau_H2 1]  ContinuousStateAttributes='p_H2'
  p_H2O : TransferFcn  Numerator=[1/K_H2O]  Denominator=[tau_H2O 1]  ContinuousStateAttributes='p_H2'
  p_O2 : TransferFcn  Numerator=[1/K_O2]  Denominator=[tau_O2 1]  ContinuousStateAttributes='p_O2'
  theta*Eid : Gain  Gain=theta
  E : Outport
  pH2FC [Pa] : Outport  Port=2
  pO2FC [Pa] : Outport  Port=3
  wires:
  n_airFC [mol/s]/1 -> n_O2in/1
  p_H2/1 -> Sum4/1
  p_O2/1 -> Sum3/2
  pH2 in/1 -> Sum4/2
  pO2in/1 -> Sum3/1
  Sum3/1 -> average air pressure/1
  Sum4/1 -> average H2 pressure/1
  p_H2O/1 -> Sum7/1
  pH2Oin/1 -> Sum7/2
  Sqrt/1 -> Product/2
  Gain/1 -> Sum1/2
  E0 [V]/1 -> Sum1/1
  Sum1/1 -> theta*Eid/1
  log/1 -> Gain/1
  Product/1 -> log/1
  theta*Eid/1 -> E/1
  atm --> Pa1/1 -> pO2FC [Pa]/1, Sqrt/1
  atm --> Pa2/1 -> Product/3
  Sum7/1 -> average H2O pressure/1
  atm --> Pa/1 -> pH2FC [Pa]/1, Product/1
  T [K]/1 -> E0 [V]/1
  average air pressure/1 -> atm --> Pa/1
  average H2 pressure/1 -> atm --> Pa1/1
  average H2O pressure/1 -> atm --> Pa2/1
  I [A]/1 -> Kr*I/1, 2*Kr*I/1
  Kr*I/1 -> Sum2/2
  n_O2in/1 -> Sum2/1
  Sum2/1 -> p_O2/1
  Sum5/1 -> p_H2/1
  n_H2FC [mol/s]/1 -> Sum5/1
  2*Kr*I/1 -> Sum6/1, Sum5/2
  n_H2OFC [mol/s]/1 -> Sum6/2
  Sum6/1 -> p_H2O/1

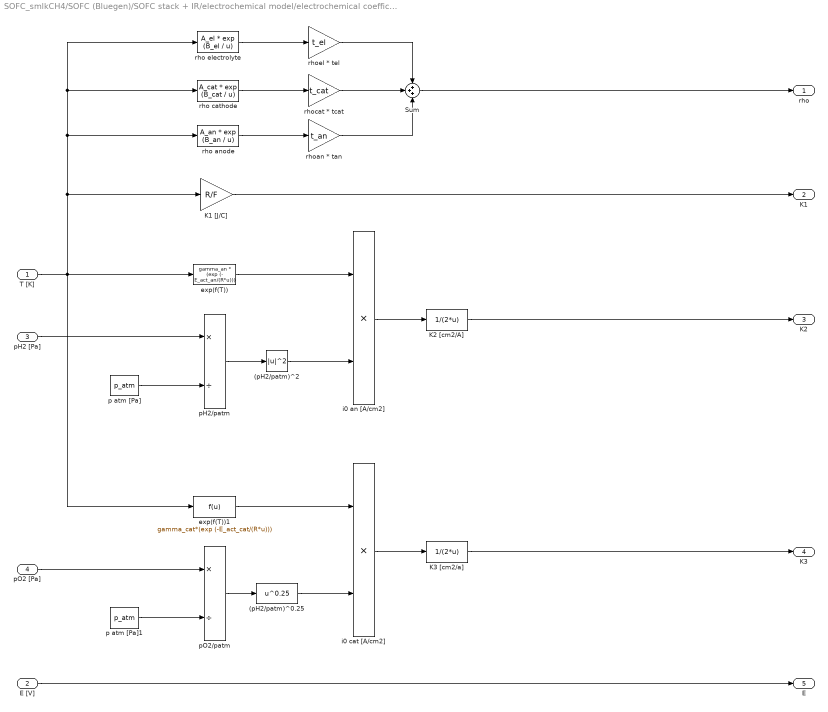
== system SOFC_smlkCH4/SOFC (Bluegen)/SOFC stack + IR/electrochemical model/electrochemical coefficients ==
  T [K] : Inport
  E [V] : Inport  Port=2
  "pH2 [Pa] " : Inport  Port=3
  pO2 [Pa] : Inport  Port=4
  (pH2/patm)^0.25 : Fcn  Expr=u^0.25
  (pH2/patm)^2 : Math  Operator=magnitude^2  SaturateOnIntegerOverflow=on
  K1 [J/C] : Gain  Gain=R/F
  K2 [cm2/A] : Fcn  Expr=1/(2*u)
  K3 [cm2/a] : Fcn  Expr=1/(2*u)
  Sum : Sum  Inputs=+++
  exp(f(T)) : Fcn  Expr=gamma_an * (exp (- E_act_an/(R*u)))
  exp(f(T))1 : Fcn  Expr=gamma_cat*(exp (-E_act_cat/(R*u)))
  i0 an [A/cm2] : Product
  i0 cat [A/cm2] : Product
  p atm [Pa] : Constant  Value=p_atm
  p atm [Pa]1 : Constant  Value=p_atm
  pH2/patm : Product  Inputs=*/
  pO2/patm : Product  Inputs=*/
  rho anode : Fcn  Expr=A_an * exp (B_an / u)
  rho cathode : Fcn  Expr=A_cat * exp (B_cat / u)
  rho electrolyte : Fcn  Expr=A_el * exp (B_el / u)
  rhoan * tan : Gain  Gain=t_an
  rhocat * tcat : Gain  Gain=t_cat
  rhoel * tel : Gain  Gain=t_el
  rho : Outport
  K1 : Outport  Port=2
  K2 : Outport  Port=3
  K3 : Outport  Port=4
  E : Outport  Port=5
  wires:
  "pH2 [Pa] "/1 -> pH2/patm/1
  p atm [Pa]/1 -> pH2/patm/2
  pH2/patm/1 -> (pH2/patm)^2/1
  T [K]/1 -> rho electrolyte/1, rho cathode/1, rho anode/1, K1 [J/C]/1, exp(f(T))1/1, exp(f(T))/1
  exp(f(T))/1 -> i0 an [A/cm2]/1
  (pH2/patm)^2/1 -> i0 an [A/cm2]/2
  p atm [Pa]1/1 -> pO2/patm/2
  pO2 [Pa]/1 -> pO2/patm/1
  pO2/patm/1 -> (pH2/patm)^0.25/1
  (pH2/patm)^0.25/1 -> i0 cat [A/cm2]/2
  exp(f(T))1/1 -> i0 cat [A/cm2]/1
  i0 an [A/cm2]/1 -> K2 [cm2/A]/1
  i0 cat [A/cm2]/1 -> K3 [cm2/a]/1
  rho electrolyte/1 -> rhoel * tel/1
  rho cathode/1 -> rhocat * tcat/1
  rho anode/1 -> rhoan * tan/1
  rhocat * tcat/1 -> Sum/2
  rhoan * tan/1 -> Sum/3
  rhoel * tel/1 -> Sum/1
  Sum/1 -> rho/1
  K1 [J/C]/1 -> K1/1
  K2 [cm2/A]/1 -> K2/1
  K3 [cm2/a]/1 -> K3/1
  E [V]/1 -> E/1

== system SOFC_smlkCH4/SOFC (Bluegen)/SOFC stack + IR/electrochemical model/internal reformer ==
  nCH4FC [mol/s] : Inport
  Constant : Constant  Value=Q_COref
  QCH4ref [W] : Gain  Gain=h_CH4ref*y_CH4
  Sum : Sum  Inputs=|++
  fuel reformer transfer function (all inclusive) : TransferFcn  Denominator=[(tau1_ref*tau2_ref) (tau1_ref+tau2_ref) 1]  ContinuousStateAttributes='q_H2'
  nH2FC : Gain  Gain=CV
  nH2OFC : Gain  Gain=CV_H2O
  nH2FC_ [mol/s] : Outport
  n_H2OFC_ [mol/s] : Outport  Port=2
  Qref [W] : Outport  Port=3
  wires:
  nCH4FC [mol/s]/1 -> fuel reformer transfer function (all inclusive)/1
  fuel reformer transfer function (all inclusive)/1 -> nH2FC/1, nH2OFC/1, QCH4ref [W]/1
  nH2FC/1 -> nH2FC_ [mol/s]/1
  nH2OFC/1 -> n_H2OFC_ [mol/s]/1
  QCH4ref [W]/1 -> Sum/1
  Constant/1 -> Sum/2
  Sum/1 -> Qref [W]/1

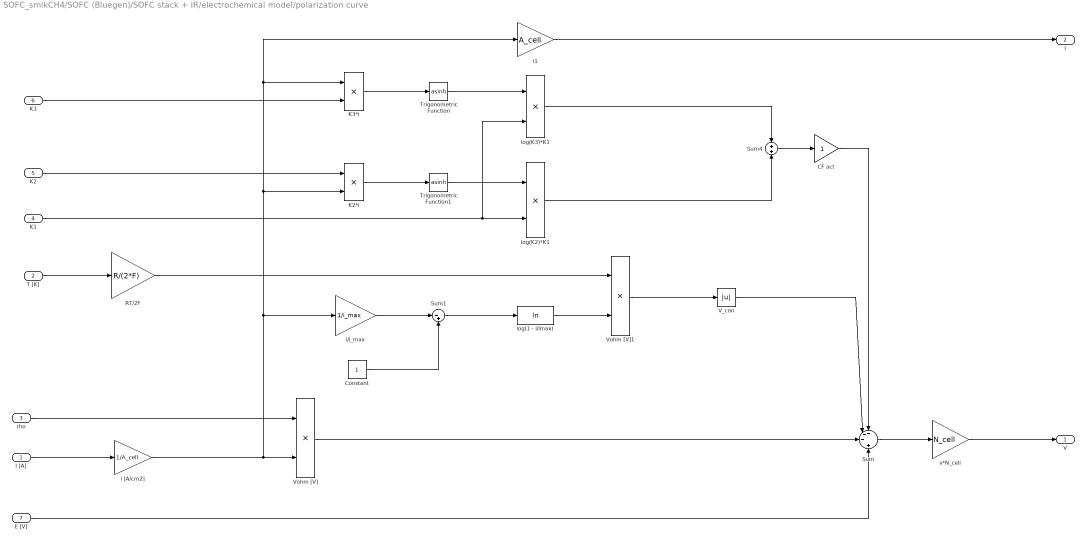
== system SOFC_smlkCH4/SOFC (Bluegen)/SOFC stack + IR/electrochemical model/polarization curve ==
  "I [A] " : Inport
  T [K] : Inport  Port=2
  rho : Inport  Port=3
  K1 : Inport  Port=4
  K2 : Inport  Port=5
  K3 : Inport  Port=6
  E [V] : Inport  Port=7
  CF act : Gain
  Constant : Constant
  K2*i : Product
  K3*i : Product
  RT/2F : Gain  Gain=R/(2*F)
  Sum : Sum  Inputs=---|+
  Sum1 : Sum  Inputs=|-+
  Sum4 : Sum  Inputs=+|+
  Trigonometric Function : Trigonometry  Operator=asinh
  Trigonometric Function1 : Trigonometry  Operator=asinh
  V_con : Abs
  Vohm [V] : Product
  Vohm [V]1 : Product
  i [A/cm2] : Gain  Gain=1/A_cell
  i/i_max : Gain  Gain=1/i_max
  i1 : Gain  Gain=A_cell
  log(1 - i/imax) : Math  Operator=log  SaturateOnIntegerOverflow=on
  log(K2)*K1 : Product
  log(K3)*K1 : Product
  v*N_cell : Gain  Gain=N_cell
  V : Outport
  I : Outport  Port=2
  wires:
  Vohm [V]/1 -> Sum/3
  v*N_cell/1 -> V/1
  "I [A] "/1 -> i [A/cm2]/1
  Sum/1 -> v*N_cell/1
  Vohm [V]1/1 -> V_con/1
  K2*i/1 -> Trigonometric Function1/1
  K3*i/1 -> Trigonometric Function/1
  Trigonometric Function1/1 -> log(K2)*K1/1
  Trigonometric Function/1 -> log(K3)*K1/1
  log(K2)*K1/1 -> Sum4/2
  log(K3)*K1/1 -> Sum4/1
  Sum4/1 -> CF act/1
  i [A/cm2]/1 -> K3*i/1, i1/1, K2*i/2, i/i_max/1, Vohm [V]/2
  Sum1/1 -> log(1 - i/imax)/1
  log(1 - i/imax)/1 -> Vohm [V]1/2
  i1/1 -> I/1
  V_con/1 -> Sum/2
  E [V]/1 -> Sum/4
  rho/1 -> Vohm [V]/1
  T [K]/1 -> RT/2F/1
  RT/2F/1 -> Vohm [V]1/1
  i/i_max/1 -> Sum1/1
  Constant/1 -> Sum1/2
  K2/1 -> K2*i/1
  K1/1 -> log(K3)*K1/2, log(K2)*K1/2
  K3/1 -> K3*i/2
  CF act/1 -> Sum/1
